simulink model "IEEE33BusTestSystem_DG"  (R2019a)
settings: Solver=VariableStepAuto  StartTime=0.0  StopTime=5  FixedStep=5e-5  RelTol=1e-3
values from neighbouring files (symbols this model uses):
  Tp = 500e-3    (= 0.5)    [IEEE33BusSystem.m]    (also in Kimc_d1_sce1-0.mat = 0.05; Kimc_d1_sce1-1.mat = 0.05; Kimc_d1_sce1-2.mat = 0.05; Kimc_d1_sce1-3.mat = 0.05)
  Tq = 50e-3    (= 0.05)    [IEEE33BusSystem.m]    (also in Kimc_d1_sce1-0.mat; Kimc_d1_sce1-1.mat; Kimc_d1_sce1-2.mat; Kimc_d1_sce1-3.mat)
libraries: powerlib x159, powerlib_meascontrol x33
(part 1 of 3)
settings Model: Creator=JY Wong  LastModifiedBy=Pablo-NB
settings DataIOCC: ReturnWorkspaceOutputs=off
settings DebuggingCC: PregeneratedLibrarySubsystemCodeDiagnostic=none  ArithmeticOperatorsInVariantConditions=warning
settings SFSimCC: SimUseLocalCustomCode=off
settings RTWCC: RTWUseLocalCustomCode=off
settings SimscapeCC: SimscapeNormalizeSystem=off

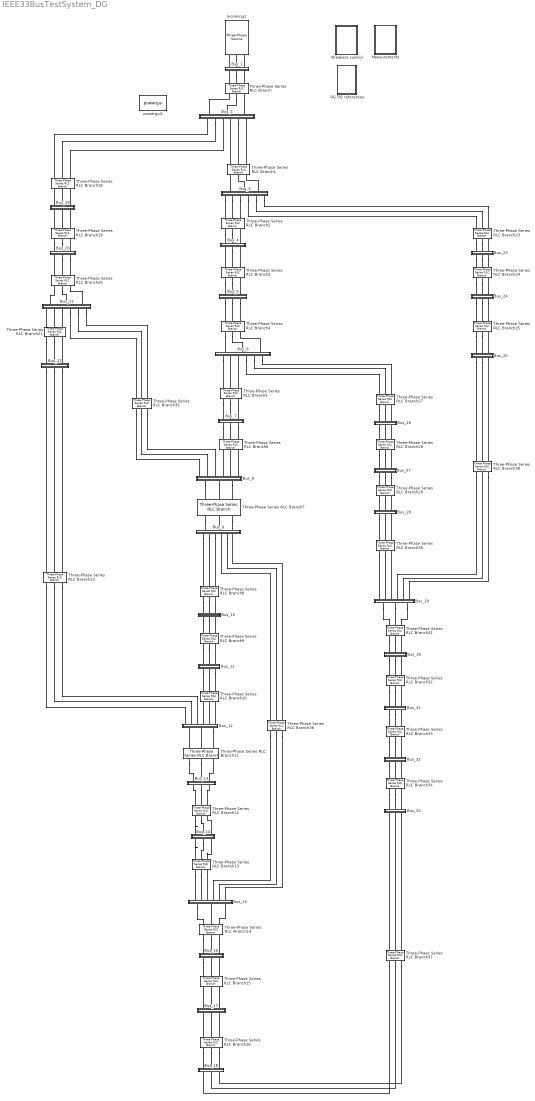
== system IEEE33BusTestSystem_DG ==
  Breakers control : Subsystem
  Bus_1 : Subsystem
  Bus_10 : Subsystem
  Bus_11 : Subsystem
  Bus_12 : Subsystem
  Bus_13 : Subsystem
  Bus_14 : Subsystem
  Bus_15 : Subsystem
  Bus_16 : Subsystem
  Bus_17 : Subsystem
  Bus_18 : Subsystem
  Bus_19 : Subsystem
  Bus_2 : Subsystem
  Bus_20 : Subsystem
  Bus_21 : Subsystem
  Bus_22 : Subsystem
  Bus_23 : Subsystem
  Bus_24 : Subsystem
  Bus_25 : Subsystem
  Bus_26 : Subsystem
  Bus_27 : Subsystem
  Bus_28 : Subsystem
  Bus_29 : Subsystem
  Bus_3 : Subsystem
  Bus_30 : Subsystem
  Bus_31 : Subsystem
  Bus_32 : Subsystem
  Bus_33 : Subsystem
  Bus_4 : Subsystem
  Bus_5 : Subsystem
  Bus_6 : Subsystem
  Bus_7 : Subsystem
  Bus_8 : Subsystem
  Bus_9 : Subsystem
  DG PQ references : Subsystem
  Incoming1 : powerlib/Electrical Sources/Three-Phase Source  InternalConnection=Yg  VoltagePhases=off  Voltage=(12660)*1  PhaseAngle=0  Voltage_phases=[25e3 25e3 25e3]/sqrt(3)  PhaseAngles_phases=[0 -120 +120]  Frequency=50  NonIdealSource=off  SpecifyImpedance=on  Resistance=0.8929  Inductance=16.58e-3  ShortCircuitLevel=438.555e6  BaseVoltage=12.66e3  XRratio=7  BusType=swing  Pref=0  Qref=0  Prefabc=[10e3, 10e3, 10e3]  Qrefabc=[0, 0, 0]  Qmin=-inf  Qmax=inf
      settings: SourceProductName=Simscape Electrical
  Measurements : Subsystem
  Three-Phase Series RLC Branch : powerlib/Elements/Three-Phase Series RLC Branch  LConnTagsString=A|B|C  RConnTagsString=A|B|C  BranchType=RL  Resistance=0.0922  Inductance=0.0470/2/pi/50  Capacitance=1e-6  Measurements=None
      settings: SourceProductName=Simscape Electrical
  Three-Phase Series RLC Branch1 : powerlib/Elements/Three-Phase Series RLC Branch  LConnTagsString=A|B|C  RConnTagsString=A|B|C  BranchType=RL  Resistance=0.4930  Inductance=0.2511/2/pi/50  Capacitance=1e-6  Measurements=None
      settings: SourceProductName=Simscape Electrical
  Three-Phase Series RLC Branch10 : powerlib/Elements/Three-Phase Series RLC Branch  LConnTagsString=A|B|C  RConnTagsString=A|B|C  BranchType=RL  Resistance=0.3744  Inductance=0.1238/2/pi/50  Capacitance=1e-6  Measurements=None
      settings: SourceProductName=Simscape Electrical
  Three-Phase Series RLC Branch11 : powerlib/Elements/Three-Phase Series RLC Branch  LConnTagsString=A|B|C  RConnTagsString=A|B|C  BranchType=RL  Resistance=1.468  Inductance=1.155/2/pi/50  Capacitance=1e-6  Measurements=None
      settings: SourceProductName=Simscape Electrical
  Three-Phase Series RLC Branch12 : powerlib/Elements/Three-Phase Series RLC Branch  LConnTagsString=A|B|C  RConnTagsString=A|B|C  BranchType=RL  Resistance=0.5416  Inductance=0.7129/2/pi/50  Capacitance=1e-6  Measurements=None
      settings: SourceProductName=Simscape Electrical
  Three-Phase Series RLC Branch13 : powerlib/Elements/Three-Phase Series RLC Branch  LConnTagsString=A|B|C  RConnTagsString=A|B|C  BranchType=RL  Resistance=0.591  Inductance=0.526/2/pi/50  Capacitance=1e-6  Measurements=None
      settings: SourceProductName=Simscape Electrical
  Three-Phase Series RLC Branch14 : powerlib/Elements/Three-Phase Series RLC Branch  LConnTagsString=A|B|C  RConnTagsString=A|B|C  BranchType=RL  Resistance=0.7463  Inductance=0.545/2/pi/50  Capacitance=1e-6  Measurements=None
      settings: SourceProductName=Simscape Electrical
  Three-Phase Series RLC Branch15 : powerlib/Elements/Three-Phase Series RLC Branch  LConnTagsString=A|B|C  RConnTagsString=A|B|C  BranchType=RL  Resistance=1.289  Inductance=1.721/2/pi/50  Capacitance=1e-6  Measurements=None
      settings: SourceProductName=Simscape Electrical
  Three-Phase Series RLC Branch16 : powerlib/Elements/Three-Phase Series RLC Branch  LConnTagsString=A|B|C  RConnTagsString=A|B|C  BranchType=RL  Resistance=0.7320  Inductance=0.5740/2/pi/50  Capacitance=1e-6  Measurements=None
      settings: SourceProductName=Simscape Electrical
  Three-Phase Series RLC Branch18 : powerlib/Elements/Three-Phase Series RLC Branch  LConnTagsString=A|B|C  RConnTagsString=A|B|C  BranchType=RL  Resistance=0.164  Inductance=0.1565/2/pi/50  Capacitance=1e-6  Measurements=None
      settings: SourceProductName=Simscape Electrical
  Three-Phase Series RLC Branch19 : powerlib/Elements/Three-Phase Series RLC Branch  LConnTagsString=A|B|C  RConnTagsString=A|B|C  BranchType=RL  Resistance=1.5042  Inductance=1.3554/2/pi/50  Capacitance=1e-6  Measurements=None
      settings: SourceProductName=Simscape Electrical
  Three-Phase Series RLC Branch2 : powerlib/Elements/Three-Phase Series RLC Branch  LConnTagsString=A|B|C  RConnTagsString=A|B|C  BranchType=RL  Resistance=0.366  Inductance=0.1864/2/pi/50  Capacitance=1e-6  Measurements=None
      settings: SourceProductName=Simscape Electrical
  Three-Phase Series RLC Branch20 : powerlib/Elements/Three-Phase Series RLC Branch  LConnTagsString=A|B|C  RConnTagsString=A|B|C  BranchType=RL  Resistance=0.4095  Inductance=0.4784/2/pi/50  Capacitance=1e-6  Measurements=None
      settings: SourceProductName=Simscape Electrical
  Three-Phase Series RLC Branch21 : powerlib/Elements/Three-Phase Series RLC Branch  LConnTagsString=A|B|C  RConnTagsString=A|B|C  BranchType=RL  Resistance=0.7089  Inductance=0.9373/2/pi/50  Capacitance=1e-6  Measurements=None
      settings: SourceProductName=Simscape Electrical
  Three-Phase Series RLC Branch22 : powerlib/Elements/Three-Phase Series RLC Branch  LConnTagsString=A|B|C  RConnTagsString=A|B|C  BranchType=RL  Resistance=2  Inductance=2/2/pi/50  Capacitance=1e-6  Measurements=None
      settings: SourceProductName=Simscape Electrical
  Three-Phase Series RLC Branch23 : powerlib/Elements/Three-Phase Series RLC Branch  LConnTagsString=A|B|C  RConnTagsString=A|B|C  BranchType=RL  Resistance=0.4512  Inductance=0.3083/2/pi/50  Capacitance=1e-6  Measurements=None
      settings: SourceProductName=Simscape Electrical
  Three-Phase Series RLC Branch24 : powerlib/Elements/Three-Phase Series RLC Branch  LConnTagsString=A|B|C  RConnTagsString=A|B|C  BranchType=RL  Resistance=0.8980  Inductance=0.7091/2/pi/50  Capacitance=1e-6  Measurements=None
      settings: SourceProductName=Simscape Electrical
  Three-Phase Series RLC Branch25 : powerlib/Elements/Three-Phase Series RLC Branch  LConnTagsString=A|B|C  RConnTagsString=A|B|C  BranchType=RL  Resistance=0.896  Inductance=0.7011/2/pi/50  Capacitance=1e-6  Measurements=None
      settings: SourceProductName=Simscape Electrical
  Three-Phase Series RLC Branch27 : powerlib/Elements/Three-Phase Series RLC Branch  LConnTagsString=A|B|C  RConnTagsString=A|B|C  BranchType=RL  Resistance=0.2030  Inductance=0.1034/2/pi/50  Capacitance=1e-6  Measurements=None
      settings: SourceProductName=Simscape Electrical
  Three-Phase Series RLC Branch28 : powerlib/Elements/Three-Phase Series RLC Branch  LConnTagsString=A|B|C  RConnTagsString=A|B|C  BranchType=RL  Resistance=0.2842  Inductance=0.1447/2/pi/50  Capacitance=1e-6  Measurements=None
      settings: SourceProductName=Simscape Electrical
  Three-Phase Series RLC Branch29 : powerlib/Elements/Three-Phase Series RLC Branch  LConnTagsString=A|B|C  RConnTagsString=A|B|C  BranchType=RL  Resistance=1.0590  Inductance=0.9337/2/pi/50  Capacitance=1e-6  Measurements=None
      settings: SourceProductName=Simscape Electrical
  Three-Phase Series RLC Branch3 : powerlib/Elements/Three-Phase Series RLC Branch  LConnTagsString=A|B|C  RConnTagsString=A|B|C  BranchType=RL  Resistance=0.3811  Inductance=0.1941/2/pi/50  Capacitance=1e-6  Measurements=None
      settings: SourceProductName=Simscape Electrical
  Three-Phase Series RLC Branch30 : powerlib/Elements/Three-Phase Series RLC Branch  LConnTagsString=A|B|C  RConnTagsString=A|B|C  BranchType=RL  Resistance=0.8042  Inductance=0.7006/2/pi/50  Capacitance=1e-6  Measurements=None
      settings: SourceProductName=Simscape Electrical
  Three-Phase Series RLC Branch31 : powerlib/Elements/Three-Phase Series RLC Branch  LConnTagsString=A|B|C  RConnTagsString=A|B|C  BranchType=RL  Resistance=0.5075  Inductance=0.2585/2/pi/50  Capacitance=1e-6  Measurements=None
      settings: SourceProductName=Simscape Electrical
  Three-Phase Series RLC Branch32 : powerlib/Elements/Three-Phase Series RLC Branch  LConnTagsString=A|B|C  RConnTagsString=A|B|C  BranchType=RL  Resistance=0.9744  Inductance=0.963/2/pi/50  Capacitance=1e-6  Measurements=None
      settings: SourceProductName=Simscape Electrical
  Three-Phase Series RLC Branch33 : powerlib/Elements/Three-Phase Series RLC Branch  LConnTagsString=A|B|C  RConnTagsString=A|B|C  BranchType=RL  Resistance=0.3105  Inductance=0.3619/2/pi/50  Capacitance=1e-6  Measurements=None
      settings: SourceProductName=Simscape Electrical
  Three-Phase Series RLC Branch34 : powerlib/Elements/Three-Phase Series RLC Branch  LConnTagsString=A|B|C  RConnTagsString=A|B|C  BranchType=RL  Resistance=0.341  Inductance=0.5302/2/pi/50  Capacitance=1e-6  Measurements=None
      settings: SourceProductName=Simscape Electrical
  Three-Phase Series RLC Branch35 : powerlib/Elements/Three-Phase Series RLC Branch  LConnTagsString=A|B|C  RConnTagsString=A|B|C  BranchType=RL  Resistance=2  Inductance=2/2/pi/50  Capacitance=1e-6  Measurements=None
      settings: SourceProductName=Simscape Electrical
  Three-Phase Series RLC Branch36 : powerlib/Elements/Three-Phase Series RLC Branch  LConnTagsString=A|B|C  RConnTagsString=A|B|C  BranchType=RL  Resistance=2  Inductance=2/2/pi/50  Capacitance=1e-6  Measurements=None
      settings: SourceProductName=Simscape Electrical
  Three-Phase Series RLC Branch37 : powerlib/Elements/Three-Phase Series RLC Branch  LConnTagsString=A|B|C  RConnTagsString=A|B|C  BranchType=RL  Resistance=0.5  Inductance=0.5/2/pi/50  Capacitance=1e-6  Measurements=None
      settings: SourceProductName=Simscape Electrical
  Three-Phase Series RLC Branch38 : powerlib/Elements/Three-Phase Series RLC Branch  LConnTagsString=A|B|C  RConnTagsString=A|B|C  BranchType=RL  Resistance=0.5  Inductance=0.5/2/pi/50  Capacitance=1e-6  Measurements=None
      settings: SourceProductName=Simscape Electrical
  Three-Phase Series RLC Branch4 : powerlib/Elements/Three-Phase Series RLC Branch  LConnTagsString=A|B|C  RConnTagsString=A|B|C  BranchType=RL  Resistance=0.819  Inductance=0.707/2/pi/50  Capacitance=1e-6  Measurements=None
      settings: SourceProductName=Simscape Electrical
  Three-Phase Series RLC Branch5 : powerlib/Elements/Three-Phase Series RLC Branch  LConnTagsString=A|B|C  RConnTagsString=A|B|C  BranchType=RL  Resistance=0.1872  Inductance=0.6188/2/pi/50  Capacitance=1e-6  Measurements=None
      settings: SourceProductName=Simscape Electrical
  Three-Phase Series RLC Branch6 : powerlib/Elements/Three-Phase Series RLC Branch  LConnTagsString=A|B|C  RConnTagsString=A|B|C  BranchType=RL  Resistance=0.7114  Inductance=0.2351/2/pi/50  Capacitance=1e-6  Measurements=None
      settings: SourceProductName=Simscape Electrical
  Three-Phase Series RLC Branch7 : powerlib/Elements/Three-Phase Series RLC Branch  LConnTagsString=A|B|C  RConnTagsString=A|B|C  BranchType=RL  Resistance=1.0300  Inductance=0.74/2/pi/50  Capacitance=1e-6  Measurements=None
      settings: SourceProductName=Simscape Electrical
  Three-Phase Series RLC Branch8 : powerlib/Elements/Three-Phase Series RLC Branch  LConnTagsString=A|B|C  RConnTagsString=A|B|C  BranchType=RL  Resistance=1.044  Inductance=0.74/2/pi/50  Capacitance=1e-6  Measurements=None
      settings: SourceProductName=Simscape Electrical
  Three-Phase Series RLC Branch9 : powerlib/Elements/Three-Phase Series RLC Branch  LConnTagsString=A|B|C  RConnTagsString=A|B|C  BranchType=RL  Resistance=0.1966  Inductance=0.065/2/pi/50  Capacitance=1e-6  Measurements=None
      settings: SourceProductName=Simscape Electrical
  powergui1 : powerlib/powergui  Priority=1  SimulationMode=Phasor  SampleTime=50e-6  frequency=50  Iterations=50  frequencyindice=50  Pbase=100e6  ErrMax=0.0001  UnitsV=kV  UnitsW=MW  buscounter=0  FunctionMessages=off  echomessages=off  EnableUseOfTLC=off  CurrentSourceSwitches=off  DisableSnubberDevices=off  DisableRonSwitches=off  DisableVfSwitches=off  DisplayEquations=off  AutomaticDiscreteSolvers=off  SolverType=Tustin/Backward Euler (TBE)  Interpol=off  ExternalGateDelay=off  methode=off  Ts=100  x0status=blocks  SPID=off  SwTol=0  HookPort=off  NonlinearTolerance=0  nMaxIteration=15  ContinueOnMaxIteration=off  RestoreLinks=warning  ResistiveCurrentMeasurement=off  Frange=[0:2:500]  Ylog=off  Xlog=on  ShowGrid=off  save=off  variable=ZData  structure=0  ZoomFFT=off  StartTime=0.0  cycles=1  DisplayStyle=1  fundamental=60  FreqAxis=off  MaxFrequency=1000  frequencyindicesteady=1  RmsSteady=2  display=off
      settings: SourceProductName=Simscape Electrical
  connections:
  Bus_1/RConn2 -- Three-Phase Series RLC Branch/LConn2
  Bus_3/RConn2 -- Three-Phase Series RLC Branch2/LConn2
  Bus_3/RConn3 -- Three-Phase Series RLC Branch2/LConn3
  Bus_3/RConn1 -- Three-Phase Series RLC Branch2/LConn1
  Bus_4/RConn2 -- Three-Phase Series RLC Branch3/LConn2
  Bus_5/RConn2 -- Three-Phase Series RLC Branch4/LConn2
  Bus_5/RConn3 -- Three-Phase Series RLC Branch4/LConn3
  Bus_5/RConn1 -- Three-Phase Series RLC Branch4/LConn1
  Three-Phase Series RLC Branch5/LConn3 -- Bus_6/RConn3
  Bus_7/RConn3 -- Three-Phase Series RLC Branch6/LConn3
  Bus_9/RConn1 -- Three-Phase Series RLC Branch8/LConn1
  Bus_19/RConn3 -- Three-Phase Series RLC Branch19/LConn3
  Bus_20/RConn3 -- Three-Phase Series RLC Branch20/LConn3
  Bus_23/RConn3 -- Three-Phase Series RLC Branch24/LConn3
  Bus_27/RConn3 -- Three-Phase Series RLC Branch29/LConn3
  Bus_27/RConn2 -- Three-Phase Series RLC Branch29/LConn2
  Three-Phase Series RLC Branch35/RConn1 -- Bus_8/LConn1
  Three-Phase Series RLC Branch35/RConn2 -- Bus_8/LConn2
  Three-Phase Series RLC Branch35/RConn3 -- Bus_8/LConn3
  Bus_3/LConn1 -- Three-Phase Series RLC Branch1/RConn1
  Bus_3/LConn2 -- Three-Phase Series RLC Branch1/RConn2
  Bus_3/LConn3 -- Three-Phase Series RLC Branch1/RConn3
  Bus_19/LConn3 -- Three-Phase Series RLC Branch18/RConn3
  Bus_19/LConn2 -- Three-Phase Series RLC Branch18/RConn2
  Bus_19/LConn1 -- Three-Phase Series RLC Branch18/RConn1
  Three-Phase Series RLC Branch19/LConn1 -- Bus_19/RConn1
  Three-Phase Series RLC Branch19/LConn2 -- Bus_19/RConn2
  Bus_20/RConn2 -- Three-Phase Series RLC Branch20/LConn2
  Bus_20/LConn3 -- Three-Phase Series RLC Branch19/RConn3
  Three-Phase Series RLC Branch19/RConn2 -- Bus_20/LConn2
  Three-Phase Series RLC Branch19/RConn1 -- Bus_20/LConn1
  Three-Phase Series RLC Branch20/LConn1 -- Bus_20/RConn1
  Three-Phase Series RLC Branch20/RConn3 -- Bus_21/LConn3
  Three-Phase Series RLC Branch20/RConn2 -- Bus_21/LConn2
  Three-Phase Series RLC Branch20/RConn1 -- Bus_21/LConn1
  Three-Phase Series RLC Branch21/LConn1 -- Bus_21/RConn1
  Three-Phase Series RLC Branch21/LConn2 -- Bus_21/RConn2
  Three-Phase Series RLC Branch21/LConn3 -- Bus_21/RConn3
  Bus_22/LConn3 -- Three-Phase Series RLC Branch21/RConn3
  Three-Phase Series RLC Branch21/RConn1 -- Bus_22/LConn1
  Bus_22/RConn1 -- Three-Phase Series RLC Branch22/LConn1
  Bus_22/RConn2 -- Three-Phase Series RLC Branch22/LConn2
  Bus_22/RConn3 -- Three-Phase Series RLC Branch22/LConn3
  Three-Phase Series RLC Branch3/LConn3 -- Bus_4/RConn3
  Bus_4/LConn3 -- Three-Phase Series RLC Branch2/RConn3
  Three-Phase Series RLC Branch2/RConn2 -- Bus_4/LConn2
  Three-Phase Series RLC Branch2/RConn1 -- Bus_4/LConn1
  Three-Phase Series RLC Branch3/LConn1 -- Bus_4/RConn1
  Bus_2/LConn3 -- Three-Phase Series RLC Branch/RConn3
  Three-Phase Series RLC Branch/RConn2 -- Bus_2/LConn2
  Bus_2/LConn1 -- Three-Phase Series RLC Branch/RConn1
  Bus_5/LConn3 -- Three-Phase Series RLC Branch3/RConn3
  Three-Phase Series RLC Branch3/RConn2 -- Bus_5/LConn2
  Three-Phase Series RLC Branch3/RConn1 -- Bus_5/LConn1
  Bus_6/LConn3 -- Three-Phase Series RLC Branch4/RConn3
  Three-Phase Series RLC Branch4/RConn2 -- Bus_6/LConn2
  Three-Phase Series RLC Branch4/RConn1 -- Bus_6/LConn1
  Bus_6/RConn1 -- Three-Phase Series RLC Branch5/LConn1
  Three-Phase Series RLC Branch5/LConn2 -- Bus_6/RConn2
  Bus_7/LConn3 -- Three-Phase Series RLC Branch5/RConn3
  Three-Phase Series RLC Branch5/RConn2 -- Bus_7/LConn2
  Three-Phase Series RLC Branch5/RConn1 -- Bus_7/LConn1
  Bus_7/RConn1 -- Three-Phase Series RLC Branch6/LConn1
  Bus_7/RConn2 -- Three-Phase Series RLC Branch6/LConn2
  Three-Phase Series RLC Branch7/RConn3 -- Bus_9/LConn3
  Bus_9/LConn2 -- Three-Phase Series RLC Branch7/RConn2
  Three-Phase Series RLC Branch7/RConn1 -- Bus_9/LConn1
  Bus_9/RConn2 -- Three-Phase Series RLC Branch8/LConn2
  Bus_9/RConn3 -- Three-Phase Series RLC Branch8/LConn3
  Bus_10/LConn3 -- Three-Phase Series RLC Branch8/RConn3
  Three-Phase Series RLC Branch8/RConn2 -- Bus_10/LConn2
  Three-Phase Series RLC Branch8/RConn1 -- Bus_10/LConn1
  Bus_10/RConn1 -- Three-Phase Series RLC Branch9/LConn1
  Bus_10/RConn2 -- Three-Phase Series RLC Branch9/LConn2
  Three-Phase Series RLC Branch9/LConn3 -- Bus_10/RConn3
  Bus_11/LConn3 -- Three-Phase Series RLC Branch9/RConn3
  Bus_11/RConn3 -- Three-Phase Series RLC Branch10/LConn3
  Three-Phase Series RLC Branch10/LConn2 -- Bus_11/RConn2
  Bus_11/RConn1 -- Three-Phase Series RLC Branch10/LConn1
  Three-Phase Series RLC Branch9/RConn1 -- Bus_11/LConn1
  Three-Phase Series RLC Branch9/RConn2 -- Bus_11/LConn2
  Bus_13/LConn3 -- Three-Phase Series RLC Branch11/RConn3
  Bus_13/RConn3 -- Three-Phase Series RLC Branch12/LConn3
  Bus_13/RConn2 -- Three-Phase Series RLC Branch12/LConn2
  Three-Phase Series RLC Branch11/RConn2 -- Bus_13/LConn2
  Three-Phase Series RLC Branch11/RConn1 -- Bus_13/LConn1
  Bus_13/RConn1 -- Three-Phase Series RLC Branch12/LConn1
  Bus_14/LConn3 -- Three-Phase Series RLC Branch12/RConn3
  Three-Phase Series RLC Branch13/LConn3 -- Bus_14/RConn3
  Three-Phase Series RLC Branch12/RConn2 -- Bus_14/LConn2
  Three-Phase Series RLC Branch12/RConn1 -- Bus_14/LConn1
  Three-Phase Series RLC Branch13/LConn1 -- Bus_14/RConn1
  Bus_14/RConn2 -- Three-Phase Series RLC Branch13/LConn2
  Bus_15/LConn3 -- Three-Phase Series RLC Branch13/RConn3
  Three-Phase Series RLC Branch13/RConn2 -- Bus_15/LConn2
  Three-Phase Series RLC Branch13/RConn1 -- Bus_15/LConn1
  Bus_16/LConn3 -- Three-Phase Series RLC Branch14/RConn3
  Three-Phase Series RLC Branch14/RConn2 -- Bus_16/LConn2
  Three-Phase Series RLC Branch14/RConn1 -- Bus_16/LConn1
  Bus_17/LConn3 -- Three-Phase Series RLC Branch15/RConn3
  Bus_17/LConn2 -- Three-Phase Series RLC Branch15/RConn2
  Bus_17/LConn1 -- Three-Phase Series RLC Branch15/RConn1
  Three-Phase Series RLC Branch16/RConn2 -- Bus_18/LConn2
  Three-Phase Series RLC Branch16/RConn1 -- Bus_18/LConn1
  Bus_23/LConn3 -- Three-Phase Series RLC Branch23/RConn3
  Three-Phase Series RLC Branch23/RConn2 -- Bus_23/LConn2
  Three-Phase Series RLC Branch23/RConn1 -- Bus_23/LConn1
  Bus_23/RConn1 -- Three-Phase Series RLC Branch24/LConn1
  Bus_23/RConn2 -- Three-Phase Series RLC Branch24/LConn2
  Bus_24/LConn3 -- Three-Phase Series RLC Branch24/RConn3
  Bus_24/RConn3 -- Three-Phase Series RLC Branch25/LConn3
  Three-Phase Series RLC Branch24/RConn2 -- Bus_24/LConn2
  Three-Phase Series RLC Branch24/RConn1 -- Bus_24/LConn1
  Bus_24/RConn2 -- Three-Phase Series RLC Branch25/LConn2
  Bus_25/LConn3 -- Three-Phase Series RLC Branch25/RConn3
  Three-Phase Series RLC Branch38/LConn3 -- Bus_25/RConn3
  Bus_25/RConn2 -- Three-Phase Series RLC Branch38/LConn2
  Bus_25/RConn1 -- Three-Phase Series RLC Branch38/LConn1
  Three-Phase Series RLC Branch25/RConn1 -- Bus_25/LConn1
  Three-Phase Series RLC Branch25/RConn2 -- Bus_25/LConn2
  Bus_26/LConn3 -- Three-Phase Series RLC Branch27/RConn3
  Three-Phase Series RLC Branch28/LConn3 -- Bus_26/RConn3
  Three-Phase Series RLC Branch27/RConn2 -- Bus_26/LConn2
  Three-Phase Series RLC Branch27/RConn1 -- Bus_26/LConn1
  Bus_26/RConn1 -- Three-Phase Series RLC Branch28/LConn1
  Bus_26/RConn2 -- Three-Phase Series RLC Branch28/LConn2
  Bus_27/LConn3 -- Three-Phase Series RLC Branch28/RConn3
  Three-Phase Series RLC Branch29/LConn1 -- Bus_27/RConn1
  Three-Phase Series RLC Branch28/RConn1 -- Bus_27/LConn1
  Three-Phase Series RLC Branch28/RConn2 -- Bus_27/LConn2
  Bus_28/LConn3 -- Three-Phase Series RLC Branch29/RConn3
  Three-Phase Series RLC Branch29/RConn2 -- Bus_28/LConn2
  Three-Phase Series RLC Branch29/RConn1 -- Bus_28/LConn1
  Three-Phase Series RLC Branch30/LConn3 -- Bus_28/RConn3
  Bus_28/RConn2 -- Three-Phase Series RLC Branch30/LConn2
  Bus_28/RConn1 -- Three-Phase Series RLC Branch30/LConn1
  Bus_29/LConn3 -- Three-Phase Series RLC Branch30/RConn3
  Three-Phase Series RLC Branch30/RConn2 -- Bus_29/LConn2
  Three-Phase Series RLC Branch30/RConn1 -- Bus_29/LConn1
  Bus_29/RConn3 -- Three-Phase Series RLC Branch31/LConn3
  Bus_29/RConn2 -- Three-Phase Series RLC Branch31/LConn2
  Bus_29/RConn1 -- Three-Phase Series RLC Branch31/LConn1
  Bus_30/LConn3 -- Three-Phase Series RLC Branch31/RConn3
  Three-Phase Series RLC Branch31/RConn2 -- Bus_30/LConn2
  Three-Phase Series RLC Branch31/RConn1 -- Bus_30/LConn1
  Bus_30/RConn3 -- Three-Phase Series RLC Branch32/LConn3
  Bus_30/RConn2 -- Three-Phase Series RLC Branch32/LConn2
  Bus_30/RConn1 -- Three-Phase Series RLC Branch32/LConn1
  Bus_31/LConn3 -- Three-Phase Series RLC Branch32/RConn3
  Three-Phase Series RLC Branch33/LConn3 -- Bus_31/RConn3
  Three-Phase Series RLC Branch32/RConn2 -- Bus_31/LConn2
  Three-Phase Series RLC Branch32/RConn1 -- Bus_31/LConn1
  Bus_31/RConn2 -- Three-Phase Series RLC Branch33/LConn2
  Bus_31/RConn1 -- Three-Phase Series RLC Branch33/LConn1
  Bus_32/LConn3 -- Three-Phase Series RLC Branch33/RConn3
  Three-Phase Series RLC Branch33/RConn2 -- Bus_32/LConn2
  Three-Phase Series RLC Branch33/RConn1 -- Bus_32/LConn1
  Three-Phase Series RLC Branch34/LConn3 -- Bus_32/RConn3
  Bus_32/RConn2 -- Three-Phase Series RLC Branch34/LConn2
  Bus_32/RConn1 -- Three-Phase Series RLC Branch34/LConn1
  Bus_33/LConn3 -- Three-Phase Series RLC Branch34/RConn3
  Three-Phase Series RLC Branch34/RConn2 -- Bus_33/LConn2
  Three-Phase Series RLC Branch34/RConn1 -- Bus_33/LConn1
  Three-Phase Series RLC Branch16/RConn3 -- Bus_18/LConn3
  Bus_1/LConn2 -- Incoming1/RConn2
  Bus_1/LConn1 -- Incoming1/RConn1
  Bus_1/LConn3 -- Incoming1/RConn3
  Three-Phase Series RLC Branch/LConn1 -- Bus_1/RConn1
  Three-Phase Series RLC Branch/LConn3 -- Bus_1/RConn3
  Bus_6/RConn4 -- Three-Phase Series RLC Branch27/LConn1
  Bus_6/RConn5 -- Three-Phase Series RLC Branch27/LConn2
  Bus_6/RConn6 -- Three-Phase Series RLC Branch27/LConn3
  Three-Phase Series RLC Branch1/LConn3 -- Bus_2/RConn6
  Bus_2/RConn5 -- Three-Phase Series RLC Branch1/LConn2
  Three-Phase Series RLC Branch1/LConn1 -- Bus_2/RConn4
  Three-Phase Series RLC Branch18/LConn3 -- Bus_2/RConn3
  Bus_2/RConn2 -- Three-Phase Series RLC Branch18/LConn2
  Three-Phase Series RLC Branch18/LConn1 -- Bus_2/RConn1
  Bus_3/RConn4 -- Three-Phase Series RLC Branch23/LConn1
  Bus_3/RConn5 -- Three-Phase Series RLC Branch23/LConn2
  Bus_3/RConn6 -- Three-Phase Series RLC Branch23/LConn3
  Bus_8/LConn6 -- Three-Phase Series RLC Branch6/RConn3
  Bus_8/LConn4 -- Three-Phase Series RLC Branch6/RConn1
  Bus_8/LConn5 -- Three-Phase Series RLC Branch6/RConn2
  Bus_8/RConn1 -- Three-Phase Series RLC Branch7/LConn1
  Three-Phase Series RLC Branch7/LConn2 -- Bus_8/RConn2
  Bus_8/RConn3 -- Three-Phase Series RLC Branch7/LConn3
  Bus_21/RConn4 -- Three-Phase Series RLC Branch35/LConn1
  Bus_21/RConn5 -- Three-Phase Series RLC Branch35/LConn2
  Bus_21/RConn6 -- Three-Phase Series RLC Branch35/LConn3
  Three-Phase Series RLC Branch21/RConn2 -- Bus_22/LConn2
  Three-Phase Series RLC Branch36/LConn1 -- Bus_9/RConn4
  Bus_9/RConn5 -- Three-Phase Series RLC Branch36/LConn2
  Three-Phase Series RLC Branch36/LConn3 -- Bus_9/RConn6
  Bus_12/LConn6 -- Three-Phase Series RLC Branch10/RConn3
  Bus_12/LConn5 -- Three-Phase Series RLC Branch10/RConn2
  Bus_12/LConn4 -- Three-Phase Series RLC Branch10/RConn1
  Three-Phase Series RLC Branch22/RConn3 -- Bus_12/LConn3
  Three-Phase Series RLC Branch22/RConn2 -- Bus_12/LConn2
  Three-Phase Series RLC Branch22/RConn1 -- Bus_12/LConn1
  Three-Phase Series RLC Branch11/LConn2 -- Bus_12/RConn2
  Three-Phase Series RLC Branch11/LConn1 -- Bus_12/RConn1
  Bus_12/RConn3 -- Three-Phase Series RLC Branch11/LConn3
  Three-Phase Series RLC Branch36/RConn1 -- Bus_15/LConn4
  Bus_15/LConn5 -- Three-Phase Series RLC Branch36/RConn2
  Three-Phase Series RLC Branch36/RConn3 -- Bus_15/LConn6
  Three-Phase Series RLC Branch14/LConn2 -- Bus_15/RConn2
  Bus_15/RConn1 -- Three-Phase Series RLC Branch14/LConn1
  Three-Phase Series RLC Branch14/LConn3 -- Bus_15/RConn3
  Three-Phase Series RLC Branch15/LConn2 -- Bus_16/RConn2
  Bus_16/RConn1 -- Three-Phase Series RLC Branch15/LConn1
  Three-Phase Series RLC Branch15/LConn3 -- Bus_16/RConn3
  Three-Phase Series RLC Branch16/LConn3 -- Bus_17/RConn3
  Three-Phase Series RLC Branch16/LConn2 -- Bus_17/RConn2
  Three-Phase Series RLC Branch16/LConn1 -- Bus_17/RConn1
  Three-Phase Series RLC Branch38/RConn1 -- Bus_29/LConn4
  Bus_29/LConn5 -- Three-Phase Series RLC Branch38/RConn2
  Three-Phase Series RLC Branch38/RConn3 -- Bus_29/LConn6
  Three-Phase Series RLC Branch37/LConn1 -- Bus_33/RConn1
  Three-Phase Series RLC Branch37/LConn2 -- Bus_33/RConn2
  Three-Phase Series RLC Branch37/LConn3 -- Bus_33/RConn3
  Three-Phase Series RLC Branch37/RConn1 -- Bus_18/RConn1
  Three-Phase Series RLC Branch37/RConn2 -- Bus_18/RConn2
  Three-Phase Series RLC Branch37/RConn3 -- Bus_18/RConn3
  Bus_24/RConn1 -- Three-Phase Series RLC Branch25/LConn1

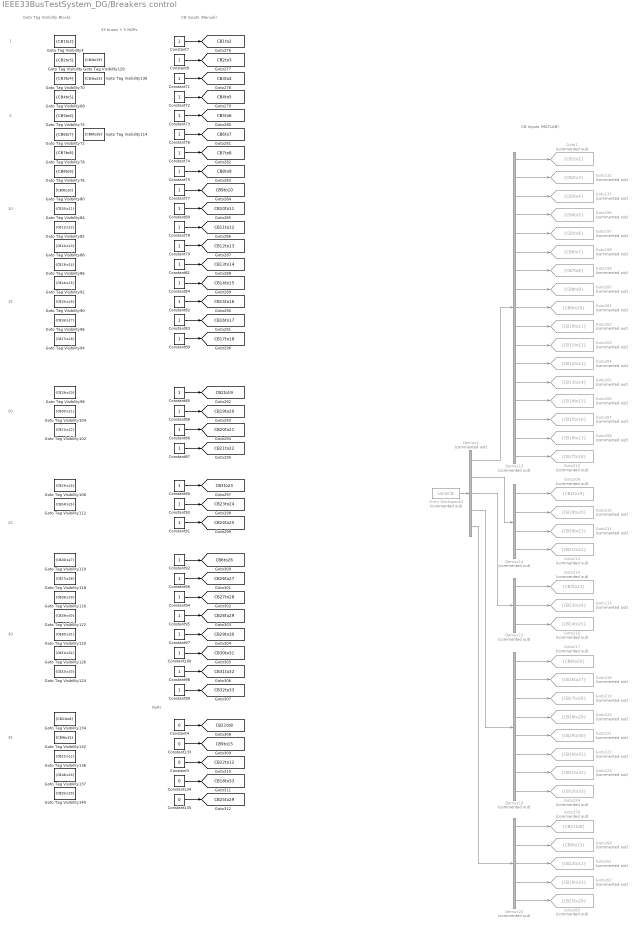
== system IEEE33BusTestSystem_DG/Breakers control ==
  note: NoPs
  note: 33 buses + 5 NOPs
  note: Goto Tag Visibility Blocks
  note: 1
  note: 5
  note: 10
  note: 15
  note: 20
  note: 25
  note: 30
  note: CB Inputs (Manual)
  note: 35
  note: CB Inputs (MATLAB)
  Constant{7..8,71..100} (32 alike) : Constant
  Constant{3..4,133..135} (5 alike) : Constant  Value=0
  Demux1 : Demux  Commented=on  Outputs=[17,4,3,8,5]
  Demux13 : Demux  Commented=on  Outputs=17
  Demux14 : Demux  Commented=on
  Demux15 : Demux  Commented=on  Outputs=3
  Demux16 : Demux  Commented=on  Outputs=8
  Demux20 : Demux  Commented=on  Outputs=5
  From Workspace1 : FromWorkspace  Commented=on  VariableName=siminCB  SampleTime=0
  Goto Tag Visibility : GotoTagVisibility  GotoTag=CB2to3
  Goto Tag Visibility102 : GotoTagVisibility  GotoTag=CB21to22
  Goto Tag Visibility104 : GotoTagVisibility  GotoTag=CB20to21
  Goto Tag Visibility106 : GotoTagVisibility  GotoTag=CB23to24
  Goto Tag Visibility110 : GotoTagVisibility  GotoTag=CB26to27
  Goto Tag Visibility112 : GotoTagVisibility  GotoTag=CB24to25
  Goto Tag Visibility114 : GotoTagVisibility  GotoTag=CB6to26
  Goto Tag Visibility116 : GotoTagVisibility  GotoTag=CB28to29
  Goto Tag Visibility118 : GotoTagVisibility  GotoTag=CB27to28
  Goto Tag Visibility120 : GotoTagVisibility  GotoTag=CB30to31
  Goto Tag Visibility122 : GotoTagVisibility  GotoTag=CB29to30
  Goto Tag Visibility124 : GotoTagVisibility  GotoTag=CB32to33
  Goto Tag Visibility126 : GotoTagVisibility  GotoTag=CB31to32
  Goto Tag Visibility129 : GotoTagVisibility  GotoTag=CB2to19
  Goto Tag Visibility130 : GotoTagVisibility  GotoTag=CB3to23
  Goto Tag Visibility132 : GotoTagVisibility  GotoTag=CB9to15
  Goto Tag Visibility134 : GotoTagVisibility  GotoTag=CB21to8
  Goto Tag Visibility136 : GotoTagVisibility  GotoTag=CB22to12
  Goto Tag Visibility137 : GotoTagVisibility  GotoTag=CB18to33
  Goto Tag Visibility140 : GotoTagVisibility  GotoTag=CB25to29
  Goto Tag Visibility4 : GotoTagVisibility  GotoTag=CB1to2
  Goto Tag Visibility68 : GotoTagVisibility  GotoTag=CB4to5
  Goto Tag Visibility70 : GotoTagVisibility  GotoTag=CB3to4
  Goto Tag Visibility72 : GotoTagVisibility  GotoTag=CB6to7
  Goto Tag Visibility74 : GotoTagVisibility  GotoTag=CB5to6
  Goto Tag Visibility76 : GotoTagVisibility  GotoTag=CB8to9
  Goto Tag Visibility78 : GotoTagVisibility  GotoTag=CB7to8
  Goto Tag Visibility80 : GotoTagVisibility  GotoTag=CB9to10
  Goto Tag Visibility82 : GotoTagVisibility  GotoTag=CB11to12
  Goto Tag Visibility84 : GotoTagVisibility  GotoTag=CB10to11
  Goto Tag Visibility86 : GotoTagVisibility  GotoTag=CB13to14
  Goto Tag Visibility88 : GotoTagVisibility  GotoTag=CB12to13
  Goto Tag Visibility90 : GotoTagVisibility  GotoTag=CB15to16
  Goto Tag Visibility92 : GotoTagVisibility  GotoTag=CB14to15
  Goto Tag Visibility94 : GotoTagVisibility  GotoTag=CB17to18
  Goto Tag Visibility96 : GotoTagVisibility  GotoTag=CB16to17
  Goto Tag Visibility98 : GotoTagVisibility  GotoTag=CB19to20
  Goto1 : Goto  Commented=on  GotoTag=CB1to2  TagVisibility=scoped
  Goto132 : Goto  Commented=on  GotoTag=CB2to3  TagVisibility=scoped
  Goto133 : Goto  Commented=on  GotoTag=CB3to4  TagVisibility=scoped
  Goto196 : Goto  Commented=on  GotoTag=CB4to5  TagVisibility=scoped
  Goto197 : Goto  Commented=on  GotoTag=CB5to6  TagVisibility=scoped
  Goto198 : Goto  Commented=on  GotoTag=CB6to7  TagVisibility=scoped
  Goto199 : Goto  Commented=on  GotoTag=CB7to8  TagVisibility=scoped
  Goto200 : Goto  Commented=on  GotoTag=CB8to9  TagVisibility=scoped
  Goto201 : Goto  Commented=on  GotoTag=CB9to10  TagVisibility=scoped
  Goto202 : Goto  Commented=on  GotoTag=CB10to11  TagVisibility=scoped
  Goto203 : Goto  Commented=on  GotoTag=CB11to12  TagVisibility=scoped
  Goto204 : Goto  Commented=on  GotoTag=CB12to13  TagVisibility=scoped
  Goto205 : Goto  Commented=on  GotoTag=CB13to14  TagVisibility=scoped
  Goto206 : Goto  Commented=on  GotoTag=CB14to15  TagVisibility=scoped
  Goto207 : Goto  Commented=on  GotoTag=CB15to16  TagVisibility=scoped
  Goto208 : Goto  Commented=on  GotoTag=CB16to17  TagVisibility=scoped
  Goto209 : Goto  Commented=on  GotoTag=CB2to19  TagVisibility=scoped
  Goto210 : Goto  Commented=on  GotoTag=CB19to20  TagVisibility=scoped
  Goto211 : Goto  Commented=on  GotoTag=CB20to21  TagVisibility=scoped
  Goto212 : Goto  Commented=on  GotoTag=CB21to22  TagVisibility=scoped
  Goto213 : Goto  Commented=on  GotoTag=CB17to18  TagVisibility=scoped
  Goto214 : Goto  Commented=on  GotoTag=CB3to23  TagVisibility=scoped
  Goto215 : Goto  Commented=on  GotoTag=CB23to24  TagVisibility=scoped
  Goto216 : Goto  Commented=on  GotoTag=CB24to25  TagVisibility=scoped
  Goto217 : Goto  Commented=on  GotoTag=CB6to26  TagVisibility=scoped
  Goto218 : Goto  Commented=on  GotoTag=CB26to27  TagVisibility=scoped
  Goto219 : Goto  Commented=on  GotoTag=CB27to28  TagVisibility=scoped
  Goto220 : Goto  Commented=on  GotoTag=CB28to29  TagVisibility=scoped
  Goto221 : Goto  Commented=on  GotoTag=CB29to30  TagVisibility=scoped
  Goto222 : Goto  Commented=on  GotoTag=CB30to31  TagVisibility=scoped
  Goto223 : Goto  Commented=on  GotoTag=CB31to32  TagVisibility=scoped
  Goto224 : Goto  Commented=on  GotoTag=CB32to33  TagVisibility=scoped
  Goto259 : Goto  Commented=on  GotoTag=CB21to8  TagVisibility=scoped
  Goto260 : Goto  Commented=on  GotoTag=CB9to15  TagVisibility=scoped
  Goto261 : Goto  Commented=on  GotoTag=CB22to12  TagVisibility=scoped
  Goto262 : Goto  Commented=on  GotoTag=CB18to33  TagVisibility=scoped
  Goto263 : Goto  Commented=on  GotoTag=CB25to29  TagVisibility=scoped
  tag scope: CB10to11=global, CB11to12=global, CB12to13=global, CB13to14=global, CB14to15=global, CB15to16=global, CB16to17=global, CB17to18=global, CB18to33=global, CB19to20=global, CB1to2=global, CB20to21=global, CB21to22=global, CB21to8=global, CB22to12=global, CB23to24=global, CB24to25=global, CB25to29=global, CB26to27=global, CB27to28=global, CB28to29=global, CB29to30=global, CB2to19=global, CB2to3=global, CB30to31=global, CB31to32=global, CB32to33=global, CB3to23=global, CB3to4=global, CB4to5=global, CB5to6=global, CB6to26=global, CB6to7=global, CB7to8=global, CB8to9=global, CB9to10=global, CB9to15=global
  wires:
  Constant72/1 -> [CB4to5]
  Constant88/1 -> [CB19to20]
  Constant93/1 -> [CB23to24]
  Constant7/1 -> [CB1to2]
  Constant76/1 -> [CB6to7]
  Constant85/1 -> [CB2to19]
  Constant75/1 -> [CB8to9]
  Constant95/1 -> [CB28to29]
  Constant73/1 -> [CB5to6]
  Constant82/1 -> [CB15to16]
  Constant96/1 -> [CB26to27]
  Constant74/1 -> [CB7to8]
  Constant91/1 -> [CB24to25]
  Constant84/1 -> [CB14to15]
  Constant100/1 -> [CB30to31]
  Constant134/1 -> [CB18to33]
  Constant99/1 -> [CB32to33]
  Constant97/1 -> [CB29to30]
  Constant81/1 -> [CB13to14]
  Constant83/1 -> [CB16to17]
  Constant8/1 -> [CB2to3]
  Constant89/1 -> [CB17to18]
  Constant98/1 -> [CB31to32]
  Constant133/1 -> [CB9to15]
  Constant4/1 -> [CB21to8]
  Constant87/1 -> [CB21to22]
  Constant94/1 -> [CB27to28]
  Constant80/1 -> [CB10to11]
  Constant79/1 -> [CB12to13]
  Constant3/1 -> [CB22to12]
  Constant90/1 -> [CB3to23]
  Constant135/1 -> [CB25to29]
  Constant92/1 -> [CB6to26]
  Constant71/1 -> [CB3to4]
  Constant78/1 -> [CB11to12]
  Constant77/1 -> [CB9to10]
  Constant86/1 -> [CB20to21]
  Demux16/2 -> Goto218/1
  Demux13/2 -> Goto132/1
  Demux14/4 -> Goto212/1
  Demux20/1 -> Goto259/1
  Demux14/1 -> Goto209/1
  Demux20/5 -> Goto263/1
  Demux16/3 -> Goto219/1
  Demux20/4 -> Goto262/1
  Demux1/5 -> Demux20/1
  Demux20/2 -> Goto260/1
  Demux15/2 -> Goto215/1
  Demux13/1 -> Goto1/1
  Demux13/6 -> Goto198/1
  Demux16/7 -> Goto223/1
  Demux20/3 -> Goto261/1
  Demux1/4 -> Demux16/1
  Demux15/1 -> Goto214/1
  Demux16/1 -> Goto217/1
  Demux1/3 -> Demux15/1
  Demux13/4 -> Goto196/1
  Demux15/3 -> Goto216/1
  Demux13/3 -> Goto133/1
  Demux16/5 -> Goto221/1
  Demux16/6 -> Goto222/1
  Demux1/2 -> Demux14/1
  Demux14/3 -> Goto211/1
  Demux13/9 -> Goto201/1
  Demux13/7 -> Goto199/1
  Demux13/13 -> Goto205/1
  Demux13/16 -> Goto208/1
  Demux16/8 -> Goto224/1
  Demux14/2 -> Goto210/1
  Demux13/12 -> Goto204/1
  Demux13/15 -> Goto207/1
  Demux13/8 -> Goto200/1
  Demux13/5 -> Goto197/1
  Demux13/17 -> Goto213/1
  Demux1/1 -> Demux13/1
  From Workspace1/1 -> Demux1/1
  Demux13/10 -> Goto202/1
  Demux16/4 -> Goto220/1
  Demux13/11 -> Goto203/1
  Demux13/14 -> Goto206/1

== system IEEE33BusTestSystem_DG/Bus_1 ==
  Bus_1 : powerlib/Measurements/Three-Phase V-I Measurement  VoltageMeasurement=phase-to-phase  SetLabelV=on  LabelV=v1_pu  Vpu=off  VpuLL=on  CurrentMeasurement=yes  SetLabelI=on  LabelI=I01_pu  Ipu=off  Pbase=100e6  Vbase=12660  OutputType=Complex  PhasorSimulation=on  PSBequivalent=0
      settings: SourceProductName=Simscape Electrical
  CB1-2 : powerlib/Elements/Three-Phase Breaker  InitialState=open  SwitchA=on  SwitchB=on  SwitchC=on  SwitchTimes="[1/60  5/60]"  External=on  BreakerResistance=0.01  SnubberResistance=1e6  SnubberCapacitance=inf  Measurements=None
      settings: SourceProductName=Simscape Electrical
  InPhaseA : PMIOPort  Side=Left
  InPhaseB : PMIOPort  Port=2  Side=Left
  InPhaseC : PMIOPort  Port=3  Side=Left
  OutPhaseA : PMIOPort  Port=4  Side=Right
  OutPhaseB : PMIOPort  Port=5  Side=Right
  OutPhaseC : PMIOPort  Port=6  Side=Right
  wires:
  [CB1to2] -> CB1-2/1
  connections:
  CB1-2/LConn1 -- Bus_1/RConn1
  CB1-2/RConn3 -- OutPhaseC/RConn1
  CB1-2/LConn2 -- Bus_1/RConn2
  CB1-2/LConn3 -- Bus_1/RConn3
  CB1-2/RConn1 -- OutPhaseA/RConn1
  CB1-2/RConn2 -- OutPhaseB/RConn1
  InPhaseA/RConn1 -- Bus_1/LConn1
  InPhaseB/RConn1 -- Bus_1/LConn2
  InPhaseC/RConn1 -- Bus_1/LConn3

== system IEEE33BusTestSystem_DG/Bus_10 ==
  Bus Load 10 : powerlib/Elements/Three-Phase Series RLC Load  LConnTagsString=A|B|C  Configuration=Y (grounded)  NominalVoltage=(12660)*0.929343  Vabc=[1e3 1e3 1e3]  Vabcp=[1e3 1e3 1e3]  NominalFrequency=50  UnbalancedPower=off  ActivePower=60e3  InductivePower=20e3  CapacitivePower=0  Pabc=[10e3 9e3 11e3]  QLabc=[100 90 110]  QCabc=[100 90 110]  Pabcp=[10e3 9e3 11e3]  QLabcp=[100 90 110]  QCabcp=[100 90 110]  Measurements=None  LoadType=constant PQ
      settings: SourceProductName=Simscape Electrical
  Bus_10 : powerlib/Measurements/Three-Phase V-I Measurement  VoltageMeasurement=phase-to-phase  SetLabelV=on  LabelV=v10_pu  Vpu=off  VpuLL=on  CurrentMeasurement=yes  SetLabelI=on  LabelI=I910_pu  Ipu=off  Pbase=100e6  Vbase=12660  OutputType=Complex  PhasorSimulation=on  PSBequivalent=0
      settings: SourceProductName=Simscape Electrical
  CB3-2 : powerlib/Elements/Three-Phase Breaker  InitialState=open  SwitchA=on  SwitchB=on  SwitchC=on  SwitchTimes="[1/60  5/60]"  External=on  BreakerResistance=0.01  SnubberResistance=1e6  SnubberCapacitance=inf  Measurements=None
      settings: SourceProductName=Simscape Electrical
  InPhaseA : PMIOPort  Side=Left
  InPhaseB : PMIOPort  Port=2  Side=Left
  InPhaseC : PMIOPort  Port=3  Side=Left
  OutPhaseA : PMIOPort  Port=4  Side=Right
  OutPhaseB : PMIOPort  Port=5  Side=Right
  OutPhaseC : PMIOPort  Port=6  Side=Right
  wires:
  [CB10to11] -> CB3-2/1
  connections:
  Bus_10/RConn1 -- CB3-2/LConn1 -- Bus Load 10/LConn1
  CB3-2/RConn3 -- OutPhaseC/RConn1
  Bus Load 10/LConn2 -- CB3-2/LConn2 -- Bus_10/RConn2
  Bus Load 10/LConn3 -- CB3-2/LConn3 -- Bus_10/RConn3
  CB3-2/RConn1 -- OutPhaseA/RConn1
  CB3-2/RConn2 -- OutPhaseB/RConn1
  InPhaseA/RConn1 -- Bus_10/LConn1
  InPhaseB/RConn1 -- Bus_10/LConn2
  InPhaseC/RConn1 -- Bus_10/LConn3

== system IEEE33BusTestSystem_DG/Bus_11 ==
  Bus Load 11 : powerlib/Elements/Three-Phase Series RLC Load  LConnTagsString=A|B|C  Configuration=Y (grounded)  NominalVoltage=(12660)*0.928485  Vabc=[1e3 1e3 1e3]  Vabcp=[1e3 1e3 1e3]  NominalFrequency=50  UnbalancedPower=off  ActivePower=45e3  InductivePower=30e3  CapacitivePower=0  Pabc=[10e3 9e3 11e3]  QLabc=[100 90 110]  QCabc=[100 90 110]  Pabcp=[10e3 9e3 11e3]  QLabcp=[100 90 110]  QCabcp=[100 90 110]  Measurements=None  LoadType=constant PQ
      settings: SourceProductName=Simscape Electrical
  Bus_11 : powerlib/Measurements/Three-Phase V-I Measurement  VoltageMeasurement=phase-to-phase  SetLabelV=on  LabelV=v11_pu  Vpu=off  VpuLL=on  CurrentMeasurement=yes  SetLabelI=on  LabelI=I1011_pu  Ipu=off  Pbase=100e6  Vbase=12660  OutputType=Complex  PhasorSimulation=on  PSBequivalent=0
      settings: SourceProductName=Simscape Electrical
  CB3-2 : powerlib/Elements/Three-Phase Breaker  InitialState=open  SwitchA=on  SwitchB=on  SwitchC=on  SwitchTimes="[1/60  5/60]"  External=on  BreakerResistance=0.01  SnubberResistance=1e6  SnubberCapacitance=inf  Measurements=None
      settings: SourceProductName=Simscape Electrical
  InPhaseA : PMIOPort  Side=Left
  InPhaseB : PMIOPort  Port=2  Side=Left
  InPhaseC : PMIOPort  Port=3  Side=Left
  OutPhaseA : PMIOPort  Port=4  Side=Right
  OutPhaseB : PMIOPort  Port=5  Side=Right
  OutPhaseC : PMIOPort  Port=6  Side=Right
  wires:
  [CB11to12] -> CB3-2/1
  connections:
  Bus_11/RConn1 -- CB3-2/LConn1 -- Bus Load 11/LConn1
  CB3-2/RConn3 -- OutPhaseC/RConn1
  Bus Load 11/LConn2 -- CB3-2/LConn2 -- Bus_11/RConn2
  Bus_11/RConn3 -- CB3-2/LConn3 -- Bus Load 11/LConn3
  CB3-2/RConn1 -- OutPhaseA/RConn1
  CB3-2/RConn2 -- OutPhaseB/RConn1
  InPhaseA/RConn1 -- Bus_11/LConn1
  InPhaseB/RConn1 -- Bus_11/LConn2
  InPhaseC/RConn1 -- Bus_11/LConn3

== system IEEE33BusTestSystem_DG/Bus_12 ==
  Bus Load 12 : powerlib/Elements/Three-Phase Series RLC Load  LConnTagsString=A|B|C  Configuration=Y (grounded)  NominalVoltage=(12660)*0.926988  Vabc=[1e3 1e3 1e3]  Vabcp=[1e3 1e3 1e3]  NominalFrequency=50  UnbalancedPower=off  ActivePower=60e3  InductivePower=35e3  CapacitivePower=0  Pabc=[10e3 9e3 11e3]  QLabc=[100 90 110]  QCabc=[100 90 110]  Pabcp=[10e3 9e3 11e3]  QLabcp=[100 90 110]  QCabcp=[100 90 110]  Measurements=None  LoadType=constant PQ
      settings: SourceProductName=Simscape Electrical
  Bus_12 : powerlib/Measurements/Three-Phase V-I Measurement  VoltageMeasurement=phase-to-phase  SetLabelV=on  LabelV=v12_pu  Vpu=off  VpuLL=on  CurrentMeasurement=yes  SetLabelI=on  LabelI=I1112_pu  Ipu=off  Pbase=100e6  Vbase=12660  OutputType=Complex  PhasorSimulation=on  PSBequivalent=0
      settings: SourceProductName=Simscape Electrical
  CB3-2 : powerlib/Elements/Three-Phase Breaker  InitialState=open  SwitchA=on  SwitchB=on  SwitchC=on  SwitchTimes="[1/60  5/60]"  External=on  BreakerResistance=0.01  SnubberResistance=1e6  SnubberCapacitance=inf  Measurements=None
      settings: SourceProductName=Simscape Electrical
  InPhaseA : PMIOPort  Side=Left
  InPhaseB : PMIOPort  Port=2  Side=Left
  InPhaseC : PMIOPort  Port=3  Side=Left
  OutPhaseA : PMIOPort  Port=4  Side=Right
  OutPhaseB : PMIOPort  Port=5  Side=Right
  OutPhaseC : PMIOPort  Port=6  Side=Right
  InPhaseA1 : PMIOPort  Port=7  Side=Left
  InPhaseB1 : PMIOPort  Port=8  Side=Left
  InPhaseC1 : PMIOPort  Port=9  Side=Left
  wires:
  [CB12to13] -> CB3-2/1
  connections:
  Bus Load 12/LConn1 -- CB3-2/LConn1 -- Bus_12/RConn1
  CB3-2/RConn3 -- OutPhaseC/RConn1
  Bus Load 12/LConn2 -- CB3-2/LConn2 -- Bus_12/RConn2
  Bus Load 12/LConn3 -- CB3-2/LConn3 -- Bus_12/RConn3
  CB3-2/RConn1 -- OutPhaseA/RConn1
  CB3-2/RConn2 -- OutPhaseB/RConn1
  InPhaseA1/RConn1 -- InPhaseA/RConn1 -- Bus_12/LConn1
  InPhaseB1/RConn1 -- InPhaseB/RConn1 -- Bus_12/LConn2
  InPhaseC1/RConn1 -- InPhaseC/RConn1 -- Bus_12/LConn3

== system IEEE33BusTestSystem_DG/Bus_13 ==
  Bus Load 13 : powerlib/Elements/Three-Phase Series RLC Load  LConnTagsString=A|B|C  Configuration=Y (grounded)  NominalVoltage=(12660)*0.920886  Vabc=[1e3 1e3 1e3]  Vabcp=[1e3 1e3 1e3]  NominalFrequency=50  UnbalancedPower=off  ActivePower=60e3  InductivePower=35e3  CapacitivePower=0  Pabc=[10e3 9e3 11e3]  QLabc=[100 90 110]  QCabc=[100 90 110]  Pabcp=[10e3 9e3 11e3]  QLabcp=[100 90 110]  QCabcp=[100 90 110]  Measurements=None  LoadType=constant PQ
      settings: SourceProductName=Simscape Electrical
  Bus_13 : powerlib/Measurements/Three-Phase V-I Measurement  VoltageMeasurement=phase-to-phase  SetLabelV=on  LabelV=v13_pu  Vpu=off  VpuLL=on  CurrentMeasurement=yes  SetLabelI=on  LabelI=I1213_pu  Ipu=off  Pbase=100e6  Vbase=12660  OutputType=Complex  PhasorSimulation=on  PSBequivalent=0
      settings: SourceProductName=Simscape Electrical
  CB3-2 : powerlib/Elements/Three-Phase Breaker  InitialState=open  SwitchA=on  SwitchB=on  SwitchC=on  SwitchTimes="[1/60  5/60]"  External=on  BreakerResistance=0.01  SnubberResistance=1e6  SnubberCapacitance=inf  Measurements=None
      settings: SourceProductName=Simscape Electrical
  InPhaseA : PMIOPort  Side=Left
  InPhaseB : PMIOPort  Port=2  Side=Left
  InPhaseC : PMIOPort  Port=3  Side=Left
  OutPhaseA : PMIOPort  Port=4  Side=Right
  OutPhaseB : PMIOPort  Port=5  Side=Right
  OutPhaseC : PMIOPort  Port=6  Side=Right
  wires:
  [CB13to14] -> CB3-2/1
  connections:
  Bus Load 13/LConn1 -- CB3-2/LConn1 -- Bus_13/RConn1
  CB3-2/RConn3 -- OutPhaseC/RConn1
  Bus Load 13/LConn2 -- CB3-2/LConn2 -- Bus_13/RConn2
  Bus_13/RConn3 -- CB3-2/LConn3 -- Bus Load 13/LConn3
  CB3-2/RConn1 -- OutPhaseA/RConn1
  CB3-2/RConn2 -- OutPhaseB/RConn1
  InPhaseB/RConn1 -- Bus_13/LConn2
  Bus_13/LConn1 -- InPhaseA/RConn1
  InPhaseC/RConn1 -- Bus_13/LConn3

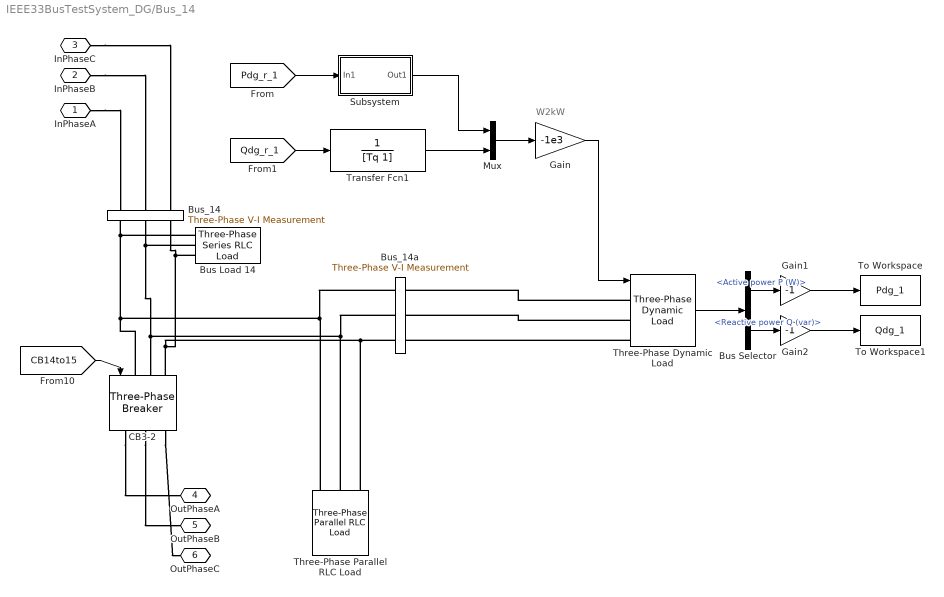
== system IEEE33BusTestSystem_DG/Bus_14 ==
  note: W2kW
  Bus Load 14 : powerlib/Elements/Three-Phase Series RLC Load  LConnTagsString=A|B|C  Configuration=Y (grounded)  NominalVoltage=(12660)*0.918624  Vabc=[1e3 1e3 1e3]  Vabcp=[1e3 1e3 1e3]  NominalFrequency=50  UnbalancedPower=off  ActivePower=120e3  InductivePower=80e3  CapacitivePower=0  Pabc=[10e3 9e3 11e3]  QLabc=[100 90 110]  QCabc=[100 90 110]  Pabcp=[10e3 9e3 11e3]  QLabcp=[100 90 110]  QCabcp=[100 90 110]  Measurements=None  LoadType=constant PQ
      settings: SourceProductName=Simscape Electrical
  Bus Selector : BusSelector  OutputSignals=Active power P (W),Reactive power Q (var)
  Bus_14 : powerlib/Measurements/Three-Phase V-I Measurement  VoltageMeasurement=phase-to-phase  SetLabelV=on  LabelV=v14_pu  Vpu=off  VpuLL=on  CurrentMeasurement=yes  SetLabelI=on  LabelI=I1314_pu  Ipu=off  Pbase=100e6  Vbase=12660  OutputType=Complex  PhasorSimulation=on  PSBequivalent=0
      settings: SourceProductName=Simscape Electrical
  Bus_14a : powerlib/Measurements/Three-Phase V-I Measurement  VoltageMeasurement=no  SetLabelV=off  LabelV=v14a_pu  Vpu=off  VpuLL=off  CurrentMeasurement=yes  SetLabelI=on  LabelI=I14a_pu  Ipu=off  Pbase=100e6  Vbase=500e3  OutputType=Complex  PhasorSimulation=on  PSBequivalent=0
      settings: SourceProductName=Simscape Electrical
  CB3-2 : powerlib/Elements/Three-Phase Breaker  InitialState=open  SwitchA=on  SwitchB=on  SwitchC=on  SwitchTimes="[1/60  5/60]"  External=on  BreakerResistance=0.01  SnubberResistance=1e6  SnubberCapacitance=inf  Measurements=None
      settings: SourceProductName=Simscape Electrical
  Gain : Gain  Gain=-1e3
  Gain1 : Gain  Gain=-1
  Gain2 : Gain  Gain=-1
  Mux : Mux  Inputs=2
  Subsystem : Subsystem
  Three-Phase Dynamic Load : powerlib/Elements/Three-Phase Dynamic Load  NominalVoltage=[ 12660 50 ]  ActiveReactivePowers=[-300 0]  PositiveSequence=[0.9348 0]  ExternalControl=on  NpNq=[1.3 2]  TimeConstants="[0  0  0  0]"  MinimumVoltage=0.7  Tfilter=1e-4  LoadFlowParameters=[4,0,0,0,0]
      settings: SourceProductName=Simscape Electrical  SourceProductBaseCode=PS
  Three-Phase Parallel RLC Load : powerlib/Elements/Three-Phase Parallel RLC Load  LConnTagsString=A|B|C  Configuration=Y (grounded)  NominalVoltage=12660  Vabc=[1e3 1e3 1e3]  Vabcp=[1e3 1e3 1e3]  NominalFrequency=50  UnbalancedPower=off  ActivePower=0.01  InductivePower=0  CapacitivePower=0  Pabc=[10e3 9e3 11e3]  QLabc=[100 90 110]  QCabc=[100 90 110]  Pabcp=[10e3 9e3 11e3]  QLabcp=[100 90 110]  QCabcp=[100 90 110]  Measurements=None  LoadType=constant Z
      settings: SourceProductName=Simscape Electrical
  To Workspace : ToWorkspace  VariableName=Pdg_1  SaveFormat=Timeseries  SampleTime=-1
  To Workspace1 : ToWorkspace  VariableName=Qdg_1  SaveFormat=Timeseries  SampleTime=-1
  Transfer Fcn1 : TransferFcn  Denominator=[Tq 1]
  InPhaseA : PMIOPort  Side=Left
  InPhaseB : PMIOPort  Port=2  Side=Left
  InPhaseC : PMIOPort  Port=3  Side=Left
  OutPhaseA : PMIOPort  Port=4  Side=Right
  OutPhaseB : PMIOPort  Port=5  Side=Right
  OutPhaseC : PMIOPort  Port=6  Side=Right
  wires:
  [CB14to15] -> CB3-2/1
  Mux/1 -> Gain/1
  Gain/1 -> Three-Phase Dynamic Load/1
  Three-Phase Dynamic Load/1 -> Bus Selector/1
  Subsystem/1(Out1) -> Mux/1
  Transfer Fcn1/1 -> Mux/2
  Bus Selector/1 -> Gain1/1  "<Active power P (W)>"
  Bus Selector/2 -> Gain2/1  "<Reactive power Q (var)>"
  Gain1/1 -> To Workspace/1
  Gain2/1 -> To Workspace1/1
  [Pdg_r_1] -> Subsystem/1(In1)
  [Qdg_r_1] -> Transfer Fcn1/1
  connections:
  CB3-2/LConn1 -- Three-Phase Parallel RLC Load/LConn1 -- Bus_14a/RConn1 -- Bus Load 14/LConn1 -- Bus_14/RConn1
  CB3-2/RConn3 -- OutPhaseC/RConn1
  Bus_14/RConn3 -- Bus_14a/RConn3 -- Three-Phase Parallel RLC Load/LConn3 -- CB3-2/LConn3 -- Bus Load 14/LConn3
  CB3-2/RConn1 -- OutPhaseA/RConn1
  CB3-2/RConn2 -- OutPhaseB/RConn1
  InPhaseB/RConn1 -- Bus_14/LConn2
  InPhaseA/RConn1 -- Bus_14/LConn1
  InPhaseC/RConn1 -- Bus_14/LConn3
  Bus_14/RConn2 -- Bus Load 14/LConn2 -- Three-Phase Parallel RLC Load/LConn2 -- Bus_14a/RConn2 -- CB3-2/LConn2
  Three-Phase Dynamic Load/LConn1 -- Bus_14a/LConn1
  Three-Phase Dynamic Load/LConn2 -- Bus_14a/LConn2
  Three-Phase Dynamic Load/LConn3 -- Bus_14a/LConn3

== system IEEE33BusTestSystem_DG/Bus_15 ==
  Bus Load 15 : powerlib/Elements/Three-Phase Series RLC Load  LConnTagsString=A|B|C  Configuration=Y (grounded)  NominalVoltage=(12660)*0.917215  Vabc=[1e3 1e3 1e3]  Vabcp=[1e3 1e3 1e3]  NominalFrequency=50  UnbalancedPower=off  ActivePower=60e3  InductivePower=10e3  CapacitivePower=0  Pabc=[10e3 9e3 11e3]  QLabc=[100 90 110]  QCabc=[100 90 110]  Pabcp=[10e3 9e3 11e3]  QLabcp=[100 90 110]  QCabcp=[100 90 110]  Measurements=None  LoadType=constant PQ
      settings: SourceProductName=Simscape Electrical
  Bus_15 : powerlib/Measurements/Three-Phase V-I Measurement  VoltageMeasurement=phase-to-phase  SetLabelV=on  LabelV=v15_pu  Vpu=off  VpuLL=on  CurrentMeasurement=yes  SetLabelI=on  LabelI=I1415_pu  Ipu=off  Pbase=100e6  Vbase=12660  OutputType=Complex  PhasorSimulation=on  PSBequivalent=0
      settings: SourceProductName=Simscape Electrical
  CB3-2 : powerlib/Elements/Three-Phase Breaker  InitialState=open  SwitchA=on  SwitchB=on  SwitchC=on  SwitchTimes="[1/60  5/60]"  External=on  BreakerResistance=0.01  SnubberResistance=1e6  SnubberCapacitance=inf  Measurements=None
      settings: SourceProductName=Simscape Electrical
  InPhaseA : PMIOPort  Side=Left
  InPhaseB : PMIOPort  Port=2  Side=Left
  InPhaseC : PMIOPort  Port=3  Side=Left
  OutPhaseA : PMIOPort  Port=4  Side=Right
  OutPhaseB : PMIOPort  Port=5  Side=Right
  OutPhaseC : PMIOPort  Port=6  Side=Right
  InPhaseA1 : PMIOPort  Port=7  Side=Left
  InPhaseB1 : PMIOPort  Port=8  Side=Left
  InPhaseC1 : PMIOPort  Port=9  Side=Left
  wires:
  [CB15to16] -> CB3-2/1
  connections:
  Bus Load 15/LConn1 -- CB3-2/LConn1 -- Bus_15/RConn1
  CB3-2/RConn3 -- OutPhaseC/RConn1
  Bus Load 15/LConn2 -- CB3-2/LConn2 -- Bus_15/RConn2
  Bus Load 15/LConn3 -- CB3-2/LConn3 -- Bus_15/RConn3
  CB3-2/RConn1 -- OutPhaseA/RConn1
  CB3-2/RConn2 -- OutPhaseB/RConn1
  InPhaseA1/RConn1 -- InPhaseA/RConn1 -- Bus_15/LConn1
  InPhaseB1/RConn1 -- InPhaseB/RConn1 -- Bus_15/LConn2
  InPhaseC1/RConn1 -- InPhaseC/RConn1 -- Bus_15/LConn3
